simulink model "mobile_wt"  (R2018a)
settings: Solver=VariableStepAuto  StartTime=0.0  StopTime=10  RelTol=1e-3
settings Model: Creator=janish  LastModifiedBy=janish

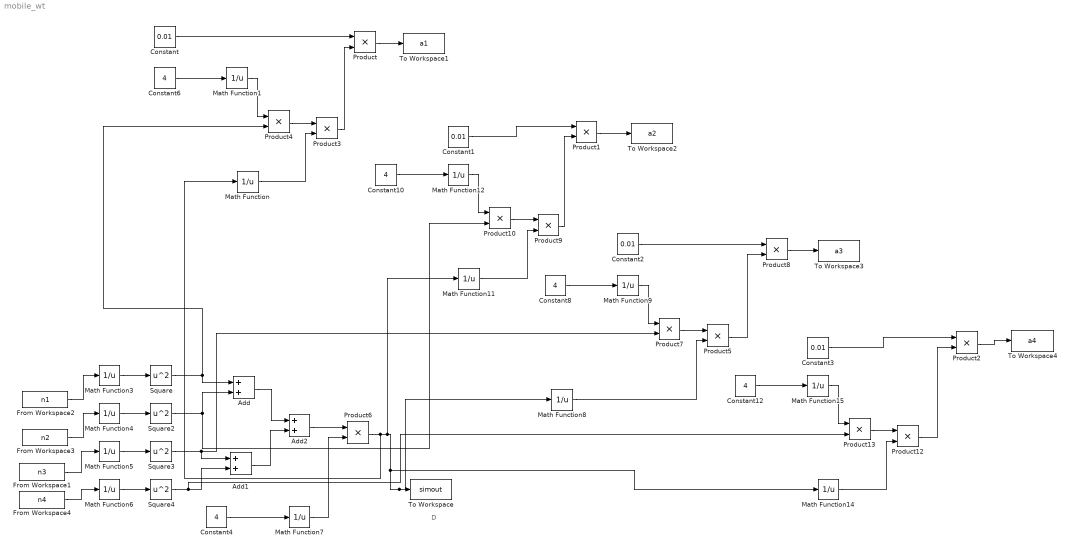
== system mobile_wt ==
  note: D
  Add : Sum
  Add1 : Sum
  Add2 : Sum
  Constant{,1..3} (4 alike) : Constant  Value=0.01
  Constant{4,6,8,10,12} (5 alike) : Constant  Value=4
  From Workspace1 : FromWorkspace  VariableName=n3  SampleTime=0
  From Workspace2 : FromWorkspace  VariableName=n1  SampleTime=0
  From Workspace3 : FromWorkspace  VariableName=n2  SampleTime=0
  From Workspace4 : FromWorkspace  VariableName=n4  SampleTime=0
  Math Function{,1,3..9,11..12,14..15} (13 alike) : Math  Operator=reciprocal  RndMeth=Zero  SaturateOnIntegerOverflow=on
  Product{,1..10,12..13} (13 alike) : Product
  Square{,2..4} (4 alike) : Math  Operator=square  SaturateOnIntegerOverflow=on
  To Workspace : ToWorkspace  VariableName=simout  SaveFormat=Timeseries  SampleTime=-1
  To Workspace1 : ToWorkspace  VariableName=a1  SampleTime=-1
      settings: Save2DSignal=2-D array (concatenate along first dimension)
  To Workspace2 : ToWorkspace  VariableName=a2  SampleTime=-1
  To Workspace3 : ToWorkspace  VariableName=a3  SampleTime=-1
  To Workspace4 : ToWorkspace  VariableName=a4  SampleTime=-1
  wires:
  Square/1 -> Product4/2, Add/1
  Product4/1 -> Product3/1
  Math Function1/1 -> Product4/1
  Math Function/1 -> Product3/2
  Constant6/1 -> Math Function1/1
  Math Function3/1 -> Square/1
  Math Function4/1 -> Square2/1
  Math Function5/1 -> Square3/1
  Math Function6/1 -> Square4/1
  Add1/1 -> Add2/2
  Add/1 -> Add2/1
  Add2/1 -> Product6/1
  Constant4/1 -> Math Function7/1
  Math Function7/1 -> Product6/2
  Product6/1 -> Math Function/1, Math Function11/1, Math Function14/1, Math Function8/1, To Workspace/1
  Square3/1 -> Product7/2, Add1/1
  Product7/1 -> Product5/1
  Math Function8/1 -> Product5/2
  Constant8/1 -> Math Function9/1
  Math Function9/1 -> Product7/1
  Square2/1 -> Product10/2, Add/2
  Product10/1 -> Product9/1
  Math Function11/1 -> Product9/2
  Constant10/1 -> Math Function12/1
  Math Function12/1 -> Product10/1
  Square4/1 -> Product13/2, Add1/2
  Product13/1 -> Product12/1
  Math Function14/1 -> Product12/2
  Constant12/1 -> Math Function15/1
  Math Function15/1 -> Product13/1
  From Workspace2/1 -> Math Function3/1
  From Workspace3/1 -> Math Function4/1
  From Workspace1/1 -> Math Function5/1
  From Workspace4/1 -> Math Function6/1
  Product12/1 -> Product2/2
  Constant3/1 -> Product2/1
  Product5/1 -> Product8/2
  Constant2/1 -> Product8/1
  Product9/1 -> Product1/2
  Constant1/1 -> Product1/1
  Constant/1 -> Product/1
  Product3/1 -> Product/2
  Product1/1 -> To Workspace2/1
  Product8/1 -> To Workspace3/1
  Product2/1 -> To Workspace4/1
  Product/1 -> To Workspace1/1
